simulink model "Arificial_potential"  (R2019a)
settings: Solver=VariableStepAuto  StartTime=0.0  StopTime=50  RelTol=1e-3
settings Model: Creator=Pranjal  LastModifiedBy=Pranjal

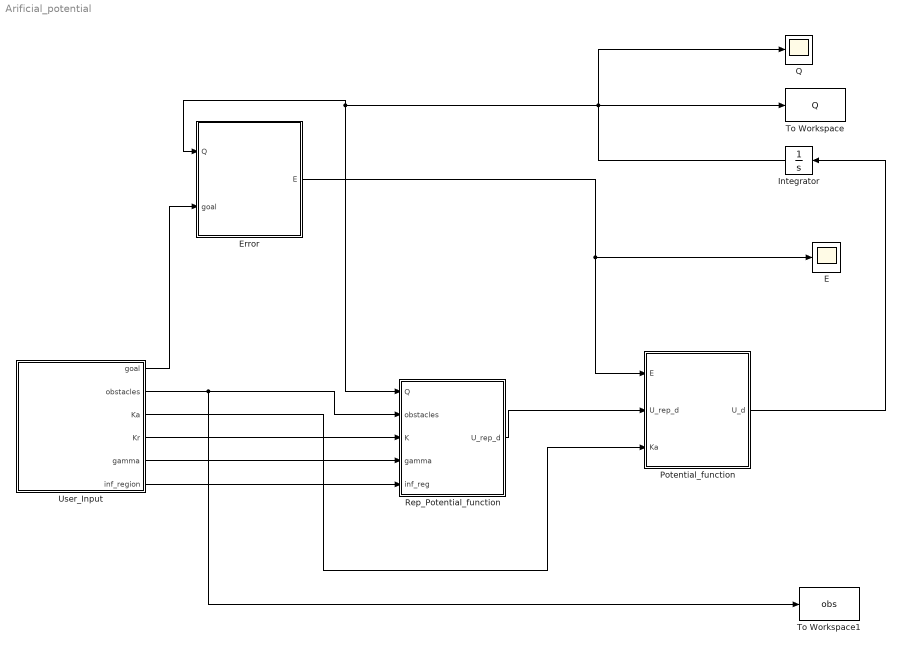
== system Arificial_potential ==
  E : Scope
  Error : MATLAB Function  TreatAsAtomicUnit=on
  Integrator : Integrator  InitialCondition=[1;1]
  Potential_function : MATLAB Function  TreatAsAtomicUnit=on
  Q : Scope
  Rep_Potential_function : MATLAB Function  TreatAsAtomicUnit=on
  To Workspace : ToWorkspace  VariableName=Q  SaveFormat=Timeseries  SampleTime=-1
  To Workspace1 : ToWorkspace  VariableName=obs  SaveFormat=Timeseries  SampleTime=-1
  User_Input : MATLAB Function  TreatAsAtomicUnit=on
  wires:
  Integrator/1 -> Q/1, Error/1(Q), Rep_Potential_function/1(Q), To Workspace/1
  User_Input/2(obstacles) -> To Workspace1/1, Rep_Potential_function/2(obstacles)
  Error/1(E) -> Potential_function/1(E), E/1
  Potential_function/1(U_d) -> Integrator/1
  User_Input/1(goal) -> Error/2(goal)
  Rep_Potential_function/1(U_rep_d) -> Potential_function/2(U_rep_d)
  User_Input/6(inf_region) -> Rep_Potential_function/5(inf_reg)
  User_Input/5(gamma) -> Rep_Potential_function/4(gamma)
  User_Input/4(Kr) -> Rep_Potential_function/3(K)
  User_Input/3(Ka) -> Potential_function/3(Ka)

== matlab function Arificial_potential/Potential_function ==
  data: E input; U_d output; U_rep_d input; Ka input
function U_d = fcn(E, U_rep_d, Ka)

U_attr_d = -Ka*E; %parabolic
% U_attr_d = -Ka*E/norm(E);%conical takes more time. So when stimulating, increase time param
U_d = U_attr_d + U_rep_d;

== matlab function Arificial_potential/User_Input ==
  data: goal output; obstacles output; Ka output; Kr output; gamma output; inf_region output
function [goal, obstacles, Ka, Kr, gamma, inf_region] = fcn()
start = [1;1];
Ka = 1;
Kr = 1;
gamma = 2;
inf_region = 2;
goal = [20;20];
obstacles = [[2 4.5 3]; %r, x, y
             [2 3 12];
             [3 15 15]];

== matlab function Arificial_potential/Error ==
  data: Q input; goal input; E output
function E = fcn(Q, goal)
E = Q - goal;

== matlab function Arificial_potential/Rep_Potential_function ==
  data: Q input; obstacles input; U_rep_d output; K input; gamma input; inf_reg input
function U_rep_d = fcn(Q, obstacles, K, gamma, inf_reg)
U_rep_d = zeros(2, 1);
for i = 1:size(obstacles, 1)
    r = obstacles(i, 1);
    c = obstacles(i, 2:3)';
    dist = norm(Q - c);
    if (dist - r) <= inf_reg
        U_rep_curr = (K*(Q - c)*(1/(dist - r) - 1/inf_reg)^(gamma - 1))/(dist*(dist - r)^2);
        U_rep_d = U_rep_d + U_rep_curr;   
    end
end
